simulink model "cub"  (R2015a)
settings: Solver=ode45  StartTime=0.0  StopTime=10.0  RelTol=1e-3
settings Model: Creator=Remy  LastModifiedBy=Remy

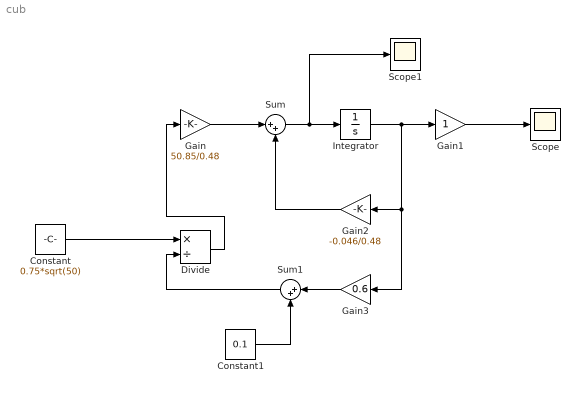
== system cub ==
  Constant : Constant  Value=0.75*sqrt(50)
  Constant1 : Constant  Value=0.1
  Divide : Product  Inputs=*/
  Gain : Gain  Gain=50.85/0.48
  Gain1 : Gain
  Gain2 : Gain  Gain=-0.046/0.48
  Gain3 : Gain  Gain=0.6
  Integrator : Integrator
  Scope : Scope
  Scope1 : Scope
  Sum : Sum  Inputs=|++
  Sum1 : Sum  Inputs=|++
  wires:
  Divide/1 -> Gain/1
  Gain/1 -> Sum/1
  Sum/1 -> Scope1/1, Integrator/1
  Integrator/1 -> Gain3/1, Gain2/1, Gain1/1
  Gain1/1 -> Scope/1
  Gain2/1 -> Sum/2
  Constant/1 -> Divide/1
  Gain3/1 -> Sum1/1
  Constant1/1 -> Sum1/2
  Sum1/1 -> Divide/2
